simulink model "chap5_4sim"  (Simulink 3.00)
settings: Solver=ode45  StartTime=0.0  StopTime=10  RelTol=1e-3
settings Model: LastModifiedBy=liu

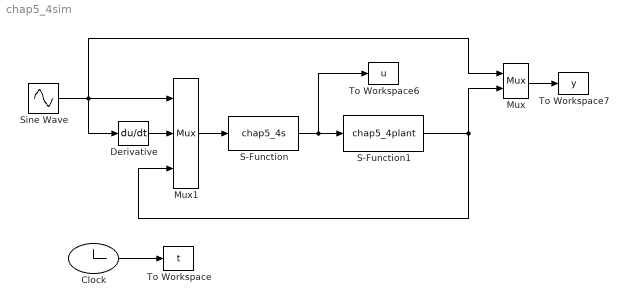
== system chap5_4sim ==
  Clock : Clock
  Derivative : Derivative
  Mux : Mux  Inputs=2
      settings: DisplayOption=none
  Mux1 : Mux  Inputs=3
      settings: DisplayOption=none
  S-Function : S-Function  FunctionName=chap5_4s  PortCounts=[]  SFunctionModules=''
  S-Function1 : S-Function  FunctionName=chap5_4plant  PortCounts=[]  SFunctionModules=''
  Sine Wave : Sin  Amplitude=1  Frequency=pi  Phase=0  SampleTime=0
  To Workspace : ToWorkspace  VariableName=t  SampleTime=-1  SaveFormat=Matrix
  To Workspace6 : ToWorkspace  VariableName=u  SampleTime=-1  SaveFormat=Matrix
  To Workspace7 : ToWorkspace  VariableName=y  SampleTime=-1  SaveFormat=Matrix
  wires:
  Mux1/1 -> S-Function/1
  Mux/1 -> To Workspace7/1
  S-Function/1 -> S-Function1/1, To Workspace6/1
  Clock/1 -> To Workspace/1
  S-Function1/1 -> Mux/2, Mux1/3
  Derivative/1 -> Mux1/2
  Sine Wave/1 -> Mux/1, Mux1/1, Derivative/1
